simulink model "rigidBodyControl"  (R2016b)
settings: Solver=VariableStepAuto  StartTime=0.0  StopTime=0.3  FixedStep=2e-4  RelTol=1e-3
values from neighbouring files (symbols this model uses):
  denG = denG{1}    [rigidBodyInit.m]
  denGc = denGc{1}    [rigidBodyInit.m]
  numG = numG{1}    [rigidBodyInit.m]
  numGc = numGc{1}    [rigidBodyInit.m]
  Ts = 1/fs    (= 0.0002)    [rigidBodyInit.m]
libraries: simulink x1, model_controller x1
settings Model: Creator=Dai Luyao  LastModifiedBy=Dai Luyao

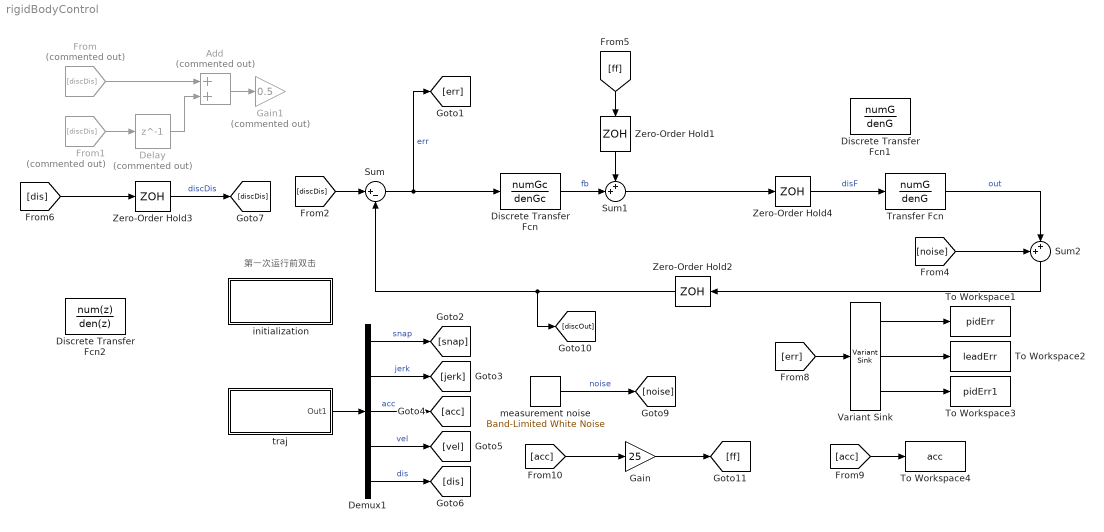
== system rigidBodyControl ==
  note: 第一次运行前双击
  Add : Sum  Commented=on
  Delay : Delay  Commented=on  DelayLength=1
  Demux1 : Demux  Outputs=5
  Discrete Transfer Fcn : DiscreteTransferFcn  Numerator=numGc  Denominator=denGc  SampleTime=Ts
  Discrete Transfer Fcn1 : DiscreteTransferFcn  Numerator=numG  Denominator=denG  SampleTime=Ts
  Discrete Transfer Fcn2 : DiscreteTransferFcn  NumeratorSource=Input port
      settings: InputPortMap=u0,p1
  From : From  Commented=on  GotoTag=discDis
  From1 : From  Commented=on  GotoTag=discDis
  Gain : Gain  Gain=25
  Gain1 : Gain  Commented=on  Gain=0.5
  Sum : Sum  Inputs=|+-
  Sum1 : Sum  Inputs=++|
  Sum2 : Sum  Inputs=++|
  To Workspace1 : ToWorkspace  VariableName=pidErr  SaveFormat=Structure With Time  SampleTime=-1
  To Workspace2 : ToWorkspace  VariableName=leadErr  SaveFormat=Structure With Time  SampleTime=-1
  To Workspace3 : ToWorkspace  VariableName=pidErr1  SaveFormat=Structure With Time  SampleTime=-1
  To Workspace4 : ToWorkspace  VariableName=acc  SaveFormat=Structure With Time  SampleTime=-1
  Transfer Fcn : TransferFcn  Numerator=numG  Denominator=denG
  Variant Sink : VariantSink
  Zero-Order Hold{1..4} (4 alike) : ZeroOrderHold  SampleTime=Ts
  initialization : Subsystem
      settings: OpenFcn=rigidBodyInit;  MoveFcn=edit rigidBodyInit;
  measurement noise : simulink/Sources/Band-Limited White Noise  Cov=noisePower  Ts=Ts  seed=[23341]
  traj : Subsystem  BlockChoice=4th order traj
      link override 3rd order traj: j=800  v=0.25  x=0.06  a=10
      settings: AttributesFormatString=%<BlockChoice>  TemplateBlock=model_controller/Profile Generators/traj  MemberBlocks=2th order traj,3rd order traj,4th order traj,step
  wires:
  Discrete Transfer Fcn/1 -> Sum1/2  "fb"
  measurement noise/1 -> [noise]  "noise"
  [noise] -> Sum2/1
  Demux1/1 -> [snap]  "snap"
  Demux1/2 -> [jerk]  "jerk"
  Demux1/3 -> [acc]  "acc"
  Demux1/4 -> [vel]  "vel"
  Demux1/5 -> [dis]  "dis"
  traj/1(Out1) -> Demux1/1
  [err] -> Variant Sink/1
  Variant Sink/1 -> To Workspace1/1
  Variant Sink/2 -> To Workspace2/1
  Variant Sink/3 -> To Workspace3/1
  [acc] -> To Workspace4/1
  Gain/1 -> [ff]
  [acc] -> Gain/1
  Sum/1 -> Discrete Transfer Fcn/1, [err]  "err"
  Zero-Order Hold3/1 -> [discDis]  "discDis"
  [dis] -> Zero-Order Hold3/1
  From1/1 -> Delay/1
  From/1 -> Add/1
  Add/1 -> Gain1/1
  Zero-Order Hold4/1 -> Transfer Fcn/1  "disF"
  [ff] -> Zero-Order Hold1/1
  Zero-Order Hold1/1 -> Sum1/1
  Sum1/1 -> Zero-Order Hold4/1
  Transfer Fcn/1 -> Sum2/2  "out"
  Sum2/1 -> Zero-Order Hold2/1
  Zero-Order Hold2/1 -> [discOut], Sum/2
  Delay/1 -> Add/2
  [discDis] -> Sum/1

== system rigidBodyControl/initialization ==

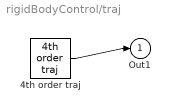
== system rigidBodyControl/traj ==
  4th order traj : model_controller/Profile Generators/4th order traj  t0=0  x=0.06  v=0.25  a=10  j=800  d=64000  Ts=0
  Out1 : Outport
  wires:
  4th order traj/1 -> Out1/1
